simulink library "robot_arms_library"  (R2020b)
settings: Solver=VariableStepAuto  StartTime=0.0  StopTime=10.0  RelTol=1e-3
libraries: nesl_utility x6, sm_lib x2
settings Model: Creator=martin  LastModifiedBy=martin

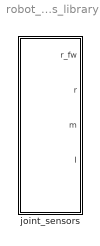
== system robot_arms_library ==
  joint_sensors : Subsystem

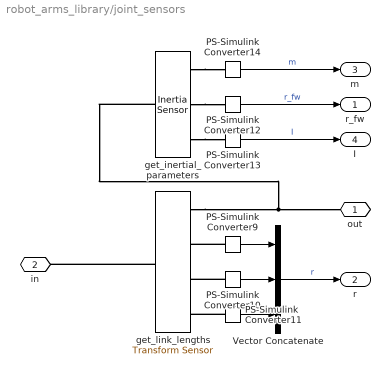
== system robot_arms_library/joint_sensors ==
  PS-Simulink Converter{9..14} (6 alike) : nesl_utility/PS-Simulink Converter  PhysicalDomain=network_engine_domain  SubClassName=ps_output  LeftPortType=input  RightPortType=output  PseudoPeriodic=off  Frequencies=[]  Unit=inherit  AffineConversion=off
  Vector Concatenate : Concatenate  NumInputs=3
  get_inertial_parameters : sm_lib/Body Elements/Inertia Sensor  SensorExtent=BodyGroup  SpanWeldJoints=off  ExcludeGroundedBodies=off  MeasurementFrame=Attached  SenseMass=on  SenseCenterOfMass=on  SenseInertiaMatrix=off  SenseCenteredInertiaMatrix=on  SensePrincipalInertiaMatrix=off  SenseRotationMatrix=off  GraphicType=PrincipalInertiaFrame  PrincipalInertiaFrameSize=20  GraphicVisPropType=SimpleVisualProperties  GraphicDiffuseColor=[0.5 0.5 0.5]  GraphicSpecularColor=[0.5 0.5 0.5 1.0]  GraphicAmbientColor=[0.15 0.15 0.15 1.0]  GraphicEmissiveColor=[0.0 0.0 0.0 1.0]  GraphicShininess=75  GraphicOpacity=1.0
      settings: SourceProductBaseCode=MS
  get_link_lengths : sm_lib/Frames and Transforms/Transform Sensor  MeasurementFrame=Follower  SenseAngle=off  SenseAxis=off  SenseAngle1=off  SenseAngle2=off  SenseAngle3=off  SenseQ=off  SenseR=off  SenseOmegaX=off  SenseOmegaY=off  SenseOmegaZ=off  SenseOmega1=off  SenseOmega2=off  SenseOmega3=off  SenseQDot=off  SenseRDot=off  SenseAlphaX=off  SenseAlphaY=off  SenseAlphaZ=off  SenseAlpha1=off  SenseAlpha2=off  SenseAlpha3=off  SenseQDDot=off  SenseRDDot=off  SenseX=on  SenseY=on  SenseZ=on  SenseRad=off  SenseAzim=off  SenseDist=off  SenseInc=off  SenseXDot=off  SenseYDot=off  SenseZDot=off  SenseRadDot=off  SenseAzimDot=off  SenseDistDot=off  SenseIncDot=off  SenseXDDot=off  SenseYDDot=off  SenseZDDot=off  SenseRadDDot=off  SenseAzimDDot=off  SenseDistDDot=off  SenseIncDDot=off
  out : PMIOPort  Side=Right
  in : PMIOPort  Port=2  Side=Left
  r_fw : Outport
  r : Outport  Port=2
  m : Outport  Port=3
  I : Outport  Port=4
  wires:
  PS-Simulink Converter11/1 -> Vector Concatenate/3
  PS-Simulink Converter9/1 -> Vector Concatenate/1
  PS-Simulink Converter14/1 -> m/1  "m"
  PS-Simulink Converter10/1 -> Vector Concatenate/2
  PS-Simulink Converter12/1 -> r_fw/1  "r_fw"
  PS-Simulink Converter13/1 -> I/1  "I"
  Vector Concatenate/1 -> r/1  "r"
  connections:
  get_inertial_parameters/RConn3 -- PS-Simulink Converter13/LConn1
  PS-Simulink Converter11/LConn1 -- get_link_lengths/RConn4
  get_inertial_parameters/RConn1 -- PS-Simulink Converter14/LConn1
  get_link_lengths/LConn1 -- in/RConn1
  get_link_lengths/RConn1 -- get_inertial_parameters/LConn1 -- out/RConn1
  PS-Simulink Converter9/LConn1 -- get_link_lengths/RConn2
  PS-Simulink Converter10/LConn1 -- get_link_lengths/RConn3
  get_inertial_parameters/RConn2 -- PS-Simulink Converter12/LConn1
